simulink model "actions"  (Simulink 7.5)
settings: Solver=FixedStepDiscrete  StartTime=0.0  StopTime=10.0  FixedStep=1  RelTol=1e-3
settings Model: Creator=vBuskirk  LastModifiedBy=C2WT
settings OptimizationCC: InitFltsAndDblsToZero=on
settings DebuggingCC: SaveWithParameterizedLinksMsg=none  StrictBusMsg=Warning
settings GRTTargetCC: TargetFcnLib=ansi_tfl_tmw.mat

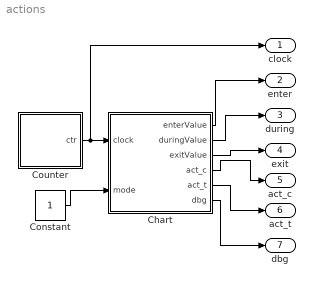
== system actions ==
  Chart : Stateflow chart  TreatAsAtomicUnit=on
  Constant : Constant  OutDataType=sfix(16)  OutScaling=2^0
  Counter : Stateflow chart  TreatAsAtomicUnit=on
  clock : Outport  OutDataType=sfix(16)  OutScaling=2^0
  enter : Outport  Port=2  OutDataType=sfix(16)  OutScaling=2^0
  during : Outport  Port=3  OutDataType=sfix(16)  OutScaling=2^0
  exit : Outport  Port=4  OutDataType=sfix(16)  OutScaling=2^0
  act_c : Outport  Port=5  OutDataType=sfix(16)  OutScaling=2^0
  act_t : Outport  Port=6  OutDataType=sfix(16)  OutScaling=2^0
  dbg : Outport  Port=7  OutDataType=sfix(16)  OutScaling=2^0
  wires:
  Chart/1(enterValue) -> enter/1
  Chart/2(duringValue) -> during/1
  Chart/3(exitValue) -> exit/1
  Chart/5(act_t) -> act_t/1
  Chart/4(act_c) -> act_c/1
  Constant/1 -> Chart/2(mode)
  Chart/6(dbg) -> dbg/1
  Counter/1(ctr) -> Chart/1(clock), clock/1

== stateflow chart Chart ==
  state M1 [parallel]
    settings: executionOrder=1
    state s1
      /*en: enterValue=1;*/
      /*du: duringValue=10+clock;*/
      /*ex: exitValue=1;*/
    state s2
      en: enterValue=2;
      du: duringValue=20+clock;
      ex: exitValue=2;
    state s3
      en: enterValue=3;
      du: duringValue=30+clock;
      ex: exitValue=3;
    s1 -> s2 : {act_c=122;}/act_t=122;
    s2 -> s3 : [clock >= 6]
        | {act_c=223;}
        | /act_t=223;
    (default) -> s1 : {act_c=21;}
        | / act_t=21;
  data: clock input double; enterValue output double =-2; duringValue output double =-3; mode input double; exitValue output double =-4; act_c output double =-5; act_t output double =-6; dbg output double =-7

== stateflow chart Counter ==
  settings: executeAtInitialization=1
  state s1
  (default) -> s1
  s1 -> s1 [order 1] : [ctr < maxVal] / ctr = ctr+1;
  s1 -> s1 [order 2] : [ctr >= maxVal] / ctr = 0;
  data: ctr output double =0; maxVal constant double =999
